simulink model "sim_2dof"  (R2023b)
settings: Solver=FixedStepAuto  StartTime=t_0  StopTime=t_f  FixedStep=dt  RelTol=1e-3
values from neighbouring files (symbols this model uses):
  C_D_lookup = sortrows(C_D_lookup, "Mach number", "ascend")    [use_simin_object.m]
undefined symbols (not defined in the file or in its folder): A_ref, C_D_brake, g, L_brake, M_dry, N_brake, v_east_0, v_up_0, W_brake, x_east_0, x_up_0
libraries: aerolibatmos2 x1, simulink x1
settings Model: Creator=Yevgeniy Gorbachev  LastModifiedBy=Yevgeniy Gorbachev
settings DataIOCC: SaveState=on  DatasetSignalFormat=timetable

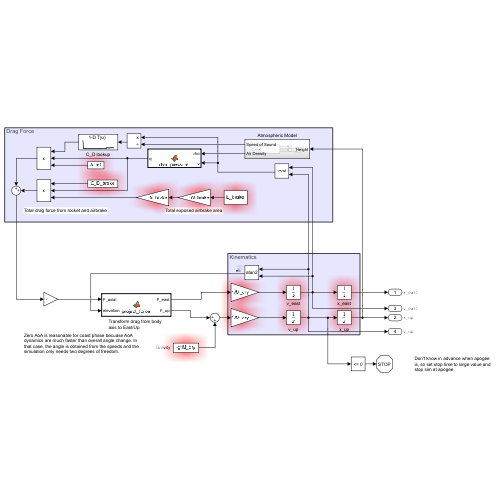
[thumbnail: Simulink's stored preview of the top-level diagram]
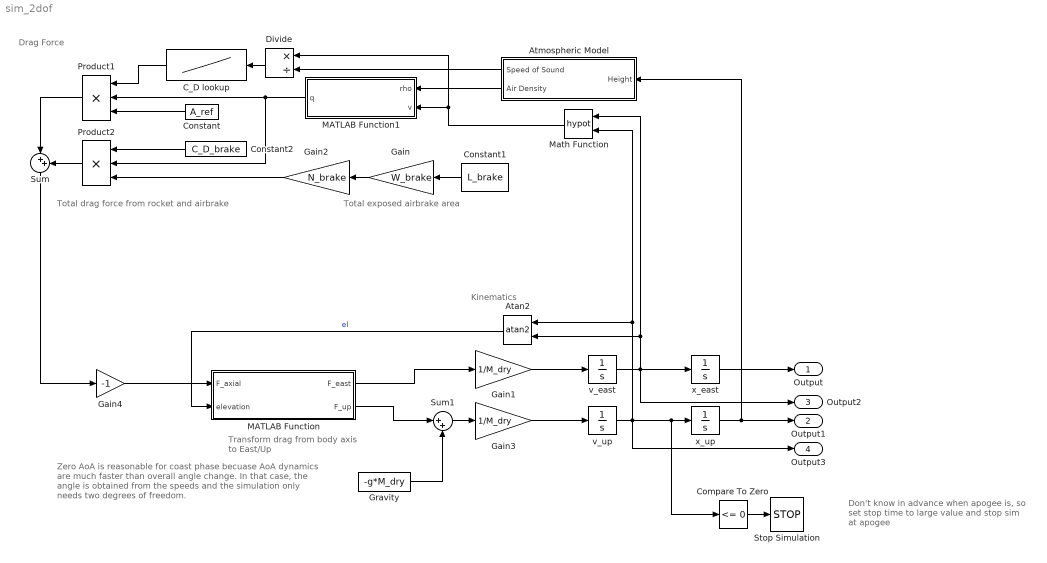
== system sim_2dof ==
  note: Total drag force from rocket and airbrake
  note: Total exposed airbrake area
  note: Kinematics
  note: Transform drag from body axis to East/Up
  note: Drag Force
  note: Zero AoA is reasonable for coast phase becuase AoA dynamics are much faster than overall angle change. In that case, the angle is obtained from the speeds and the simulation only needs two degrees of freedom.
  note: Don't know in advance when apogee is, so set stop time to large value and stop sim at apogee
  Atan2 : Trigonometry  Operator=atan2
  Atmospheric Model : Subsystem
  C_D lookup : Lookup_n-D  NumberOfTableDimensions=1  BreakpointsForDimension1="C_D_lookup.(\"Mach number\")"  Table="C_D_lookup.(\"Drag coefficient\")"  InternalRulePriority=Speed  RndMeth=Simplest
  Compare To Zero : simulink/Logic and Bit Operations/Compare To Zero  relop=<=  OutDataTypeStr=boolean
  Constant : Constant  Value=A_ref
  Constant1 : Constant  Value=L_brake
  Constant2 : Constant  Value=C_D_brake
  Divide : Product  Inputs=*/
  Gain : Gain  Gain=W_brake
  Gain1 : Gain  Gain=1/M_dry
  Gain2 : Gain  Gain=N_brake
  Gain3 : Gain  Gain=1/M_dry
  Gain4 : Gain  Gain=-1
  Gravity : Constant  Value=-g*M_dry
  MATLAB Function : MATLAB Function  TreatAsAtomicUnit=on
  MATLAB Function1 : MATLAB Function  TreatAsAtomicUnit=on
  Math Function : Math  Operator=hypot
  Product1 : Product  Inputs=3
  Product2 : Product  Inputs=3
  Stop Simulation : Stop
  Sum : Sum  Inputs=|++
  Sum1 : Sum  Inputs=|++
  v_east : Integrator  InitialCondition=v_east_0  ContinuousStateAttributes='v_east'
  v_up : Integrator  InitialCondition=v_up_0  ContinuousStateAttributes='v_east'
  x_east : Integrator  InitialCondition=x_east_0  ContinuousStateAttributes='x_up'
  x_up : Integrator  InitialCondition=x_up_0  ContinuousStateAttributes='x_up'
  Output : Outport  SignalName=x_east
  Output1 : Outport  Port=2  SignalName=x_up
  Output2 : Outport  Port=3  SignalName=v_east
  Output3 : Outport  Port=4  SignalName=v_up
  wires:
  v_up/1 -> Math Function/2, Atan2/1, Output3/1, Compare To Zero/1, x_up/1
  Gain1/1 -> v_east/1
  Gain3/1 -> v_up/1
  Compare To Zero/1 -> Stop Simulation/1
  MATLAB Function/1(F_east) -> Gain1/1
  v_east/1 -> Math Function/1, Atan2/2, Output2/1, x_east/1
  Atan2/1 -> MATLAB Function/2(elevation)  "el"
  Gravity/1 -> Sum1/2
  MATLAB Function/2(F_up) -> Sum1/1
  Sum1/1 -> Gain3/1
  x_up/1 -> Atmospheric Model/1(Height), Output1/1
  x_east/1 -> Output/1
  Math Function/1 -> MATLAB Function1/2(v), Divide/1
  MATLAB Function1/1(q) -> Product2/2, Product1/2
  Constant/1 -> Product1/3
  C_D lookup/1 -> Product1/1
  Divide/1 -> C_D lookup/1
  Atmospheric Model/1(Speed of Sound) -> Divide/2
  Atmospheric Model/2(Air Density) -> MATLAB Function1/1(rho)
  Gain4/1 -> MATLAB Function/1(F_axial)
  Sum/1 -> Gain4/1
  Product1/1 -> Sum/1
  Constant2/1 -> Product2/1
  Gain/1 -> Gain2/1
  Product2/1 -> Sum/2
  Constant1/1 -> Gain/1
  Gain2/1 -> Product2/3

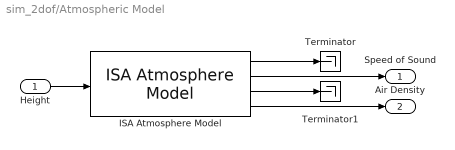
== system sim_2dof/Atmospheric Model ==
  Height : Inport
  ISA Atmosphere Model : aerolibatmos2/ISA Atmosphere Model  useExtended=off  action=Warning  custom=off  viscosityOut=off  g=9.80665  gamma=1.4  R=287.0531  L=0.0065  h_trop=11000  h_strat=20000  rho0=1.225  P0=101325  T0=288.15  h0=0
  Terminator : Terminator
  Terminator1 : Terminator
  Speed of Sound : Outport
  Air Density : Outport  Port=2
  wires:
  ISA Atmosphere Model/3 -> Terminator1/1
  ISA Atmosphere Model/1 -> Terminator/1
  ISA Atmosphere Model/4 -> Air Density/1
  Height/1 -> ISA Atmosphere Model/1
  ISA Atmosphere Model/2 -> Speed of Sound/1

== matlab function sim_2dof/MATLAB Function ==
  data: F_axial input; F_east output; elevation input; F_up output
function [F_east, F_up] = project_force(F_axial, elevation)
    F_east = F_axial*cos(elevation);
    F_up = F_axial*sin(elevation);
end

== matlab function sim_2dof/MATLAB Function1 ==
  data: rho input; v input double size=1; q output double size=1
function q = dyn_pressure(rho, v)
    q = 1/2*rho*v^2;
end
